simulink model "flow_meter"  (R2023b)
settings: Solver=VariableStepAuto  StartTime=0.0  StopTime=.1  RelTol=1e-3
libraries: simulink x2, dspsrcs4 x1, dspswit3 x1
settings Model: Creator=stark  LastModifiedBy=stark

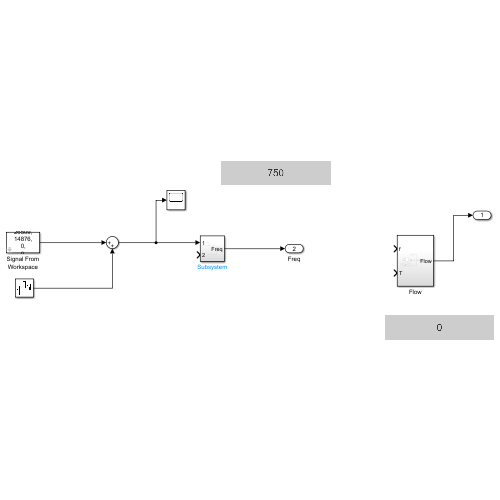
[thumbnail: Simulink's stored preview of the top-level diagram]
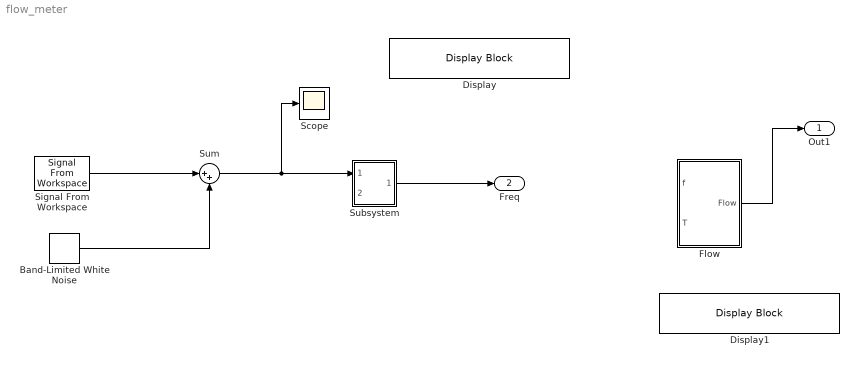
== system flow_meter ==
  Band-Limited White Noise : simulink/Sources/Band-Limited White Noise  Cov=327.67  Ts=0.1  seed=[23341]
  Display : DisplayBlock  LabelPosition=Hide  Transparency=1
  Display1 : DisplayBlock  LabelPosition=Hide  Transparency=1
  Flow : Subsystem
  Scope : Scope
  Signal From Workspace : dspsrcs4/Signal From Workspace  X=|  Ts=.0001  nsamps=1  OutputAfterFinalValue=Holding final value  ignoreOrWarnInputAndFrameLengths=off  OutputFrames=off
      | [0,
      | 14876,
      | 26509,
      | 32364,
      | 31164,
      | 23170,
      | 10126,
      | 0,
      | 0,
      | 0,
      | 0,
      | 0,
      | 0,
      | 0,
      | 10126,
      | 23170,
      | 31164,
      | 32364,
      | 26509,
      | 14876,
      | 0,
      | 0,
      | 0,
      | 0,
      | 0,
      | 0,
      | 0,
      | 5126,
      | 19260,
      | 29196,
      | 32768,
      | 29196,
      | 19260,
      | 5126,
      | 0,
      | 0,
      | 0,
      | 0,
      | 0,
      | 0,
      | 0,
      | 14876,
      | 26509,
      | 32364,
      | 31164,
      | 23170,
      | 10126,
      | 0,
      | 0,
      | 0,
      | 0,
      | 0,
      | 0,
      | 0,
      | 10126,
      | 23170,
      | 31164,
      | 32364,
      | 26509,
      | 14876,
      | 0,
      | 0,
      | 0,
      | 0,
      | 0,
      | 0,
      | 0,
      | 5126,
      | 19260,
      | 29196,
      | 32768,
      | 29196,
      | 19260,
      | 5126,
      | 0,
      | 0,
      | 0,
      | 0,
      | 0,
      | 0,
      | 0,
      | 14876,
      | 26509,
      | 32364,
      | 31164,
      | 23170,
      | 10126,
      | 0,
      | 0,
      | 0,
      | 0,
      | 0,
      | 0,
      | 0,
      | 10126,
      | 23170,
      | 31164,
      | 32364,
      | 26509,
      | 14876,
      | 0,
      | 0,
      | 0,
      | 0,
      | 0,
      | 0,
      | 0,
      | 5126,
      | 19260,
      | 29196,
      | 32768,
      | 29196,
      | 19260,
      | 5126,
      | 0,
      | 0,
      | 0,
      | 0,
      | 0,
      | 0,
      | 0,
      | 14876,
      | 26509,
      | 32364,
      | 31164,
      | 23170,
      | 10126,
      | 0,
      | 0,
      | 0,
      | 0,
      | 0,
      | 0,
      | 0,
      | 10126,
      | 23170,
      | 31164,
      | 32364,
      | 26509,
      | 14876,
      | 0,
      | 0,
      | 0,
      | 0,
      | 0,
      | 0,
      | 0,
      | 5126,
      | 19260,
      | 29196,
      | 32768,
      | 29196,
      | 19260,
      | 5126,
      | 0,
      | 0,
      | 0,
      | 0,
      | 0,
      | 0,
      | 0,
      | 14876,
      | 26509,
      | 32364,
      | 31164,
      | 23170,
      | 10126,
      | 0,
      | 0,
      | 0,
      | 0,
      | 0,
      | 0,
      | 0,
      | 10126,
      | 23170,
      | 31164,
      | 32364,
      | 26509,
      | 14876,
      | 0,
      | 0,
      | 0,
      | 0,
      | 0,
      | 0,
      | 0,
      | 5126,
      | 19260,
      | 29196,
      | 32768,
      | 29196,
      | 19260,
      | 5126,
      | 0,
      | 0,
      | 0,
      | 0,
      | 0,
      | 0,
      | 0,
      | 14876,
      | 26509,
      | 32364,
      | 31164,
      | 23170,
      | 10126,
      | 0,
      | 0,
      | 0,
      | 0,
      | 0,
      | 0,
      | 0,
      | 10126,
      | 23170,
      | 31164,
      | 32364,
      | 26509,
      | 14876,
      | 0,
      | 0,
      | 0,
      | 0,
      | 0,
      | 0,
      | 0,
      | 5126,
      | 19260,
      | 29196,
      | 32768,
      | 29196,
      | 19260,
      | 5126,
      | 0,
      | 0,
      | 0,
      | 0,
      | 0,
      | 0,
      | 0,
      | 14876,
      | 26509,
      | 32364,
      | 31164,
      | 23170,
      | 10126,
      | 0,
      | 0,
      | 0,
      | 0,
      | 0,
      | 0,
      | 0,
      | 10126,
      | 23170,
      | 31164,
      | 32364,
      | 26509,
      | 14876,
      | 0,
      | 0,
      | 0,
      | 0,
      | 0,
      | 0,
      | 0,
      | 5126,
      | 19260,
      | 29196,
      | 32768,
      | 29196,
      | 19260,
      | 5126,
      | 0,
      | 0,
      | 0,
      | 0,
      | 0,
      | 0,
      | 0,
      | 14876,
      | 26509,
      | 32364,
      | 31164,
      | 23170,
      | 10126,
      | 0,
      | 0,
      | 0,
      | 0,
      | 0,
      | 0,
      | 0,
      | 10126,
      | 23170,
      | 31164,
      | 32364,
      | 26509,
      | 14876,
      | 0,
      | 0,
      | 0,
      | 0,
      | 0,
      | 0,
      | 0,
      | 5126,
      | 19260,
      | 29196,
      | 32768,
      | 29196,
      | 19260,
      | 5126,
      | 0,
      | 0,
      | 0,
      | 0,
      | 0,
      | 0,
      | 0,
      | 14876,
      | 26509,
      | 32364,
      | 31164,
      | 23170,
      | 10126,
      | 0,
      | 0,
      | 0,
      | 0,
      | 0,
      | 0,
      | 0,
      | 10126,
      | 23170,
      | 31164,
      | 32364,
      | 26509,
      | 14876,
      | 0,
      | 0,
      | 0,
      | 0,
      | 0,
      | 0,
      | 0,
      | 5126,
      | 19260,
      | 29196,
      | 32768,
      | 29196,
      | 19260,
      | 5126,
      | 0,
      | 0,
      | 0,
      | 0,
      | 0,
      | 0,
      | 0,
      | 14876,
      | 26509,
      | 32364,
      | 31164,
      | 23170,
      | 10126,
      | 0,
      | 0,
      | 0,
      | 0,
      | 0,
      | 0,
      | 0,
      | 10126,
      | 23170,
      | 31164,
      | 32364,
      | 26509,
      | 14876,
      | 0,
      | 0,
      | 0,
      | 0,
      | 0,
      | 0,
      | 0,
      | 5126,
      | 19260,
      | 29196,
      | 32768,
      | 29196,
      | 19260,
      | 5126,
      | 0,
      | 0,
      | 0,
      | 0,
      | 0,
      | 0,
      | 0,
      | 14876,
      | 26509,
      | 32364,
      | 31164,
      | 23170,
      | 10126,
      | 0,
      | 0,
      | 0,
      | 0,
      | 0,
      | 0,
      | 0,
      | 10126,
      | 23170,
      | 31164,
      | 32364,
      | 26509,
      | 14876,
      | 0,
      | 0,
      | 0,
      | 0,
      | 0,
      | 0,
      | 0,
      | 5126,
      | 19260,
      | 29196,
      | 32768,
      | 29196,
      | 19260,
      | 5126,
      | 0,
      | 0,
      | 0,
      | 0,
      | 0,
      | 0,
      | 0,
      | 14876,
      | 26509,
      | 32364,
      | 31164,
      | 23170,
      | 10126,
      | 0,
      | 0,
      | 0,
      | 0,
      | 0,
      | 0,
      | 0,
      | 10126,
      | 23170,
      | 31164,
      | 32364,
      | 26509,
      | 14876,
      | 0,
      | 0,
      | 0,
      | 0,
      | 0,
      | 0,
      | 0,
      | 5126,
      | 19260,
      | 29196,
      | 32768,
      | 29196,
      | 19260,
      | 5126,
      | 0,
      | 0,
      | 0,
      | 0,
      | 0,
      | 0,
      | 0,
      | 14876,
      | 26509,
      | 32364,
      | 31164,
      | 23170,
      | 10126,
      | 0,
      | 0,
      | 0,
      | 0,
      | 0,
      | 0,
      | 0,
      | 10126,
      | 23170,
      | 31164,
      | 32364,
      | 26509,
      | 14876,
      | 0,
      | 0,
      | 0,
      | 0,
      | 0,
      | 0,
      | 0,
      | 5126,
      | 19260,
      | 29196,
      | 32768,
      | 29196,
      | 19260,
      | 5126,
      | 0,
      | 0,
      | 0,
      | 0,
      | 0,
      | 0,
      | 0,
      | 14876,
      | 26509,
      | 32364,
      | 31164,
      | 23170,
      | 10126,
      | 0,
      | 0,
      | 0,
      | 0,
      | 0,
      | 0,
      | 0,
      | 10126,
      | 23170,
      | 31164,
      | 32364,
      | 26509,
      | 14876,
      | 0,
      | 0,
      | 0,
      | 0,
      | 0,
      | 0,
      | 0,
      | 5126,
      | 19260,
      | 29196,
      | 32768,
      | 29196,
      | 19260,
      | 5126,
      | 0,
      | 0,
      | 0,
      | 0,
      | 0,
      | 0,
      | 0,
      | 14876,
      | 26509,
      | 32364,
      | 31164,
      | 23170,
      | 10126,
      | 0,
      | 0,
      | 0,
      | 0,
      | 0,
      | 0,
      | 0,
      | 10126,
      | 23170,
      | 31164,
      | 32364,
      | 26509,
      | 14876,
      | 0,
      | 0,
      | 0,
      | 0,
      | 0,
      | 0,
      | 0,
      | 5126,
      | 19260,
      | 29196,
      | 32768,
      | 29196,
      | 19260,
      | 5126,
      | 0,
      | 0,
      | 0,
      | 0,
      | 0,
      | 0,
      | 0,
      | 14876,
      | 26509,
      | 32364,
      | 31164,
      | 23170,
      | 10126,
      | 0,
      | 0,
      | 0,
      | 0,
      | 0,
      | 0,
      | 0,
      | 10126,
      | 23170,
      | 31164,
      | 32364,
      | 26509,
      | 14876,
      | 0,
      | 0,
      | 0,
      | 0,
      | 0,
      | 0,
      | 0,
      | 5126,
      | 19260,
      | 29196,
      | 32768,
      | 29196,
      | 19260,
      | 5126,
      | 0,
      | 0,
      | 0,
      | 0,
      | 0,
      | 0,
      | 0,
      | 14876,
      | 26509,
      | 32364,
      | 31164,
      | 23170,
      | 10126,
      | 0,
      | 0,
      | 0,
      | 0,
      | 0,
      | 0,
      | 0,
      | 10126,
      | 23170,
      | 31164,
      | 32364,
      | 26509,
      | 14876,
      | 0,
      | 0,
      | 0,
      | 0,
      | 0,
      | 0,
      | 0,
      | 5126,
      | 19260,
      | 29196,
      | 32768,
      | 29196,
      | 19260,
      | 5126,
      | 0,
      | 0,
      | 0,
      | 0,
      | 0,
      | 0,
      | 0,
      | 14876,
      | 26509,
      | 32364,
      | 31164,
      | 23170,
      | 10126,
      | 0,
      | 0,
      | 0,
      | 0,
      | 0,
      | 0,
      | 0,
      | 10126,
      | 23170,
      | 31164,
      | 32364,
      | 26509,
      | 14876,
      | 0,
      | 0,
      | 0,
      | 0,
      | 0,
      | 0,
      | 0,
      | 5126,
      | 19260,
      | 29196,
      | 32768,
      | 29196,
      | 19260,
      | 5126,
      | 0,
      | 0,
      | 0,
      | 0,
      | 0,
      | 0,
      | 0,
      | 14876,
      | 26509,
      | 32364,
      | 31164,
      | 23170,
      | 10126,
      | 0,
      | 0,
      | 0,
      | 0,
      | 0,
      | 0,
      | 0,
      | 10126,
      | 23170,
      | 31164,
      | 32364,
      | 26509,
      | 14876,
      | 0,
      | 0,
      | 0,
      | 0,
      | 0,
      | 0,
      | 0,
      | 5126,
      | 19260,
      | 29196,
      | 32768,
      | 29196,
      | 19260,
      | 5126,
      | 0,
      | 0,
      | 0,
      | 0,
      | 0,
      | 0,
      | 0,
      | 14876,
      | 26509,
      | 32364,
      | 31164,
      | 23170,
      | 10126,
      | 0,
      | 0,
      | 0,
      | 0,
      | 0,
      | 0,
      | 0,
      | 10126,
      | 23170,
      | 31164,
      | 32364,
      | 26509,
      | 14876,
      | 0,
      | 0,
      | 0,
      | 0,
      | 0,
      | 0,
      | 0,
      | 5126,
      | 19260,
      | 29196,
      | 32768,
      | 29196,
      | 19260,
      | 5126,
      | 0,
      | 0,
      | 0,
      | 0,
      | 0,
      | 0,
      | 0,
      | 14876,
      | 26509,
      | 32364,
      | 31164,
      | 23170,
      | 10126,
      | 0,
      | 0,
      | 0,
      | 0,
      | 0,
      | 0,
      | 0,
      | 10126,
      | 23170,
      | 31164,
      | 32364,
      | 26509,
      | 14876,
      | 0,
      | 0,
      | 0,
      | 0,
      | 0,
      | 0,
      | 0,
      | 5126,
      | 19260,
      | 29196,
      | 32768,
      | 29196,
      | 19260,
      | 5126,
      | 0,
      | 0,
      | 0,
      | 0,
      | 0,
      | 0,
      | 0,
      | 14876,
      | 26509,
      | 32364,
      | 31164,
      | 23170,
      | 10126,
      | 0,
      | 0,
      | 0,
      | 0,
      | 0,
      | 0,
      | 0,
      | 10126,
      | 23170,
      | 31164,
      | 32364,
      | 26509,
      | 14876,
      | 0,
      | 0,
      | 0,
      | 0,
      | 0,
      | 0,
      | 0,
      | 5126,
      | 19260,
      | 29196,
      | 32768,
      | 29196,
      | 19260,
      | 5126,
      | 0,
      | 0,
      | 0,
      | 0,
      | 0,
      | 0,
      | 0,
      | 14876,
      | 26509,
      | 32364,
      | 31164,
      | 23170,
      | 10126,
      | 0,
      | 0,
      | 0,
      | 0,
      | 0,
      | 0,
      | 0,
      | 10126,
      | 23170,
      | 31164,
      | 32364,
      | 26509,
      | 14876,
      | 0,
      | 0,
      | 0,
      | 0,
      | 0,
      | 0,
      | 0,
      | 5126,
      | 19260,
      | 29196,
      | 32768,
      | 29196,
      | 19260,
      | 5126,
      | 0,
      | 0,
      | 0,
      | 0,
      | 0,
      | 0,
      | 0,
      | 14876,
      | 26509,
      | 32364,
      | 31164,
      | 23170,
      | 10126,
      | 0,
      | 0,
      | 0,
      | 0,
      | 0,
      | 0,
      | 0,
      | 10126,
      | 23170,
      | 31164,
      | 32364,
      | 26509,
      | 14876,
      | 0,
      | 0,
      | 0,
      | 0,
      | 0,
      | 0,
      | 0,
      | 5126,
      | 19260,
      | 29196,
      | 32768,
      | 29196,
      | 19260,
      | 5126,
      | 0,
      | 0,
      | 0,
      | 0,
      | 0,
      | 0,
      | 0,
      | 14876,
      | 26509,
      | 32364,
      | 31164,
      | 23170,
      | 10126,
      | 0,
      | 0,
      | 0,
      | 0,
      | 0,
      | 0,
      | 0,
      | 10126,
      | 23170,
      | 31164,
      | 32364,
      | 26509,
      | 14876,
      | 0,
      | 0,
      | 0,
      | 0,
      | 0,
      | 0,
      | 0,
      | 5126,
      | 19260,
      | 29196,
      | 32768,
      | 29196,
      | 19260,
      | 5126,
      | 0,
      | 0,
      | 0,
      | 0,
      | 0,
      | 0]
  Subsystem : Subsystem
  Sum : Sum  Inputs=|++
  Out1 : Outport
  Freq : Outport  Port=2
  wires:
  Sum/1 -> Scope/1, Subsystem/1(In1)
  Signal From Workspace/1 -> Sum/1
  Band-Limited White Noise/1 -> Sum/2
  Flow/1(Flow) -> Out1/1
  Subsystem/1(Freq) -> Freq/1

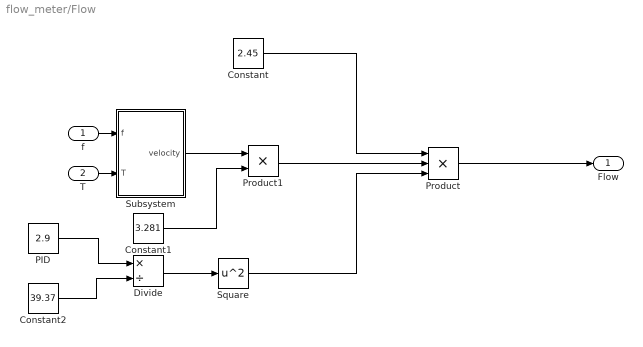
== system flow_meter/Flow ==
  f : Inport
  T : Inport  Port=2
  Constant : Constant  Value=2.45
  Constant1 : Constant  Value=3.281
  Constant2 : Constant  Value=39.37
  Divide : Product  Inputs=*/
  "PID " : Constant  Value=2.9
  Product : Product  Inputs=3
  Product1 : Product
  Square : Math  Operator=square
  Subsystem : Subsystem
  Flow : Outport
  wires:
  Constant/1 -> Product/1
  Constant2/1 -> Divide/2
  Product/1 -> Flow/1
  "PID "/1 -> Divide/1
  f/1 -> Subsystem/1(f)
  T/1 -> Subsystem/2(T)
  Divide/1 -> Square/1
  Square/1 -> Product/3
  Subsystem/1(velocity) -> Product1/1
  Product1/1 -> Product/2
  Constant1/1 -> Product1/2

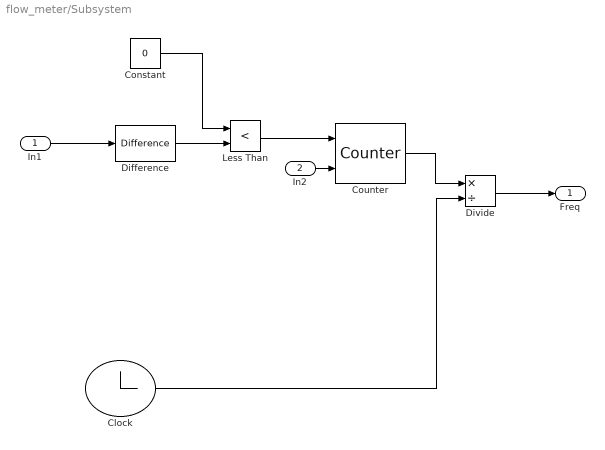
== system flow_meter/Subsystem ==
  In1 : Inport
  In2 : Inport  Port=2
  Clock : Clock
  Constant : Constant  Value=0
  Counter : dspswit3/Counter  Direction=Up  CountEvent=Rising edge  CounterSize=32 bits  MaxCount=255  InitialCount=0  Output=Count  HitValue=32  ResetInput=on  SamplesPerFrame=1  Ts=1  CntDtype=double  HitDtype=Logical
  Difference : simulink/Discrete/Difference  ICPrevInput=0.0  OutMin=[]  OutMax=[]  OutDataType=fixdt(1, 16)  OutScaling=2^-10  DoSatur=off
  Divide : Product  Inputs=*/
  Less Than : RelationalOperator  Operator=<  OutDataTypeStr=boolean  RndMeth=Simplest  InputSameDT=off
  Freq : Outport
  wires:
  Constant/1 -> Less Than/1
  Less Than/1 -> Counter/1
  Clock/1 -> Divide/2
  Divide/1 -> Freq/1
  In2/1 -> Counter/2
  Counter/1 -> Divide/1
  Difference/1 -> Less Than/2
  In1/1 -> Difference/1

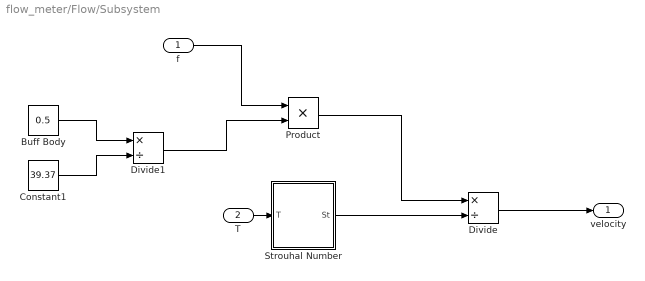
== system flow_meter/Flow/Subsystem ==
  f : Inport
  T : Inport  Port=2
  Buff Body : Constant  Value=0.5
  Constant1 : Constant  Value=39.37
  Divide : Product  Inputs=*/
  Divide1 : Product  Inputs=*/
  Product : Product
  Strouhal Number : Subsystem
  velocity : Outport
  wires:
  Product/1 -> Divide/1
  Buff Body/1 -> Divide1/1
  Strouhal Number/1(St) -> Divide/2
  f/1 -> Product/1
  Divide1/1 -> Product/2
  Constant1/1 -> Divide1/2
  Divide/1 -> velocity/1
  T/1 -> Strouhal Number/1(T)

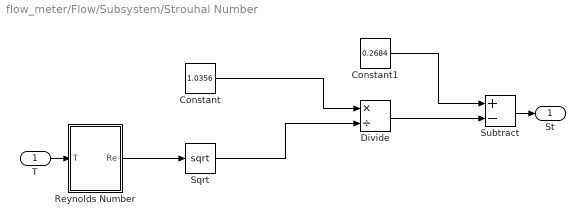
== system flow_meter/Flow/Subsystem/Strouhal Number ==
  T : Inport
  Constant : Constant  Value=1.0356
  Constant1 : Constant  Value=0.2684
  Divide : Product  Inputs=*/
  Reynolds Number : Subsystem
  Sqrt : Sqrt
  Subtract : Sum  Inputs=+-
  St : Outport
  wires:
  Subtract/1 -> St/1
  Constant1/1 -> Subtract/1
  Sqrt/1 -> Divide/2
  Reynolds Number/1(Re) -> Sqrt/1
  Divide/1 -> Subtract/2
  T/1 -> Reynolds Number/1(T)
  Constant/1 -> Divide/1

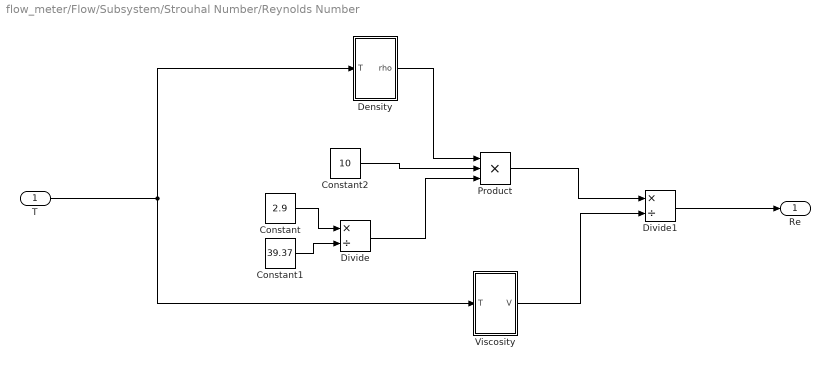
== system flow_meter/Flow/Subsystem/Strouhal Number/Reynolds Number ==
  T : Inport
  Constant : Constant  Value=2.9
  Constant1 : Constant  Value=39.37
  Constant2 : Constant  Value=10
  Density : Subsystem
  Divide : Product  Inputs=*/
  Divide1 : Product  Inputs=*/
  Product : Product  Inputs=3
  Viscosity : Subsystem
  Re : Outport
  wires:
  Product/1 -> Divide1/1
  Constant1/1 -> Divide/2
  Viscosity/1(V) -> Divide1/2
  Constant/1 -> Divide/1
  Density/1(rho) -> Product/1
  Divide1/1 -> Re/1
  Divide/1 -> Product/3
  Constant2/1 -> Product/2
  T/1 -> Density/1(T), Viscosity/1(T)

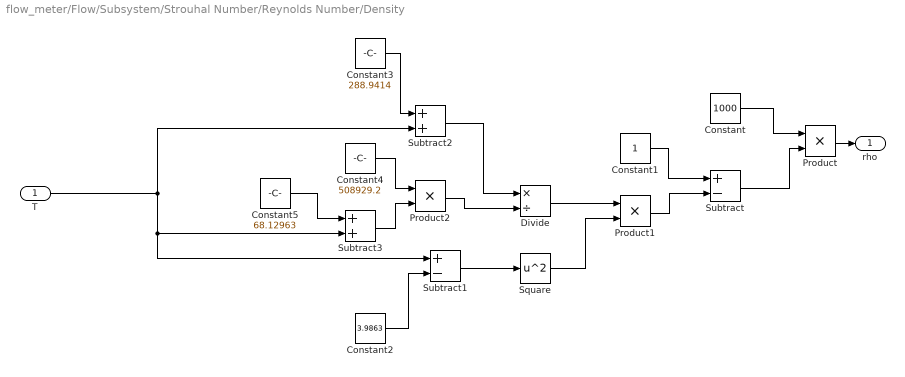
== system flow_meter/Flow/Subsystem/Strouhal Number/Reynolds Number/Density ==
  T : Inport
  Constant : Constant  Value=1000
  Constant1 : Constant
  Constant2 : Constant  Value=3.9863
  Constant3 : Constant  Value=288.9414
  Constant4 : Constant  Value=508929.2
  Constant5 : Constant  Value=68.12963
  Divide : Product  Inputs=*/
  Product : Product
  Product1 : Product
  Product2 : Product
  Square : Math  Operator=square
  Subtract : Sum  Inputs=+-
  Subtract1 : Sum  Inputs=+-
  Subtract2 : Sum
  Subtract3 : Sum
  rho : Outport
  wires:
  Constant5/1 -> Subtract3/1
  T/1 -> Subtract2/2, Subtract1/1, Subtract3/2
  Constant4/1 -> Product2/1
  Constant/1 -> Product/1
  Divide/1 -> Product1/1
  Subtract1/1 -> Square/1
  Constant1/1 -> Subtract/1
  Product/1 -> rho/1
  Constant2/1 -> Subtract1/2
  Square/1 -> Product1/2
  Subtract/1 -> Product/2
  Subtract3/1 -> Product2/2
  Product1/1 -> Subtract/2
  Product2/1 -> Divide/2
  Constant3/1 -> Subtract2/1
  Subtract2/1 -> Divide/1

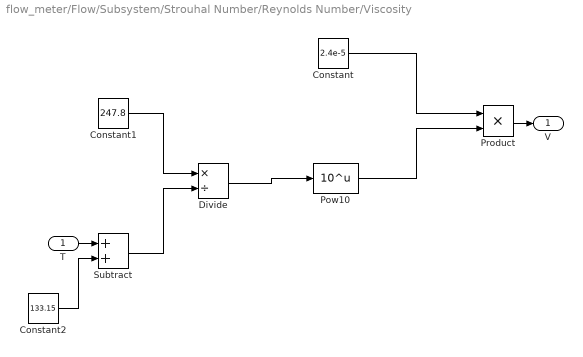
== system flow_meter/Flow/Subsystem/Strouhal Number/Reynolds Number/Viscosity ==
  T : Inport
  Constant : Constant  Value=2.4e-5
  Constant1 : Constant  Value=247.8
  Constant2 : Constant  Value=133.15
  Divide : Product  Inputs=*/
  Pow10 : Math  Operator=10^u  SignedPower=on  RndMeth=Zero
  Product : Product
  Subtract : Sum
  V : Outport
  wires:
  Constant2/1 -> Subtract/2
  Constant/1 -> Product/1
  Pow10/1 -> Product/2
  Subtract/1 -> Divide/2
  Constant1/1 -> Divide/1
  Divide/1 -> Pow10/1
  Product/1 -> V/1
  T/1 -> Subtract/1
